simulink model "calculatingcontrol"  (R2023b)
settings: Solver=VariableStepAuto  StartTime=0.0  StopTime=4  RelTol=1e-3
values from neighbouring files (symbols this model uses):
  Kd = params(3)    [ObjectiveFunction_FOPID.m]    (also in run_FOPID_Control.m = best_position_SSA(3))
  Kp = params(1)    [ObjectiveFunction_FOPID.m]    (also in run_FOPID_Control.m = best_position_SSA(1))
undefined symbols (not defined in the file or in its folder): my_gravity_torque, my_mass_matrix, my_velocity_product, q_d, qd_d
settings Model: Creator=孙伟杰  LastModifiedBy=孙伟杰

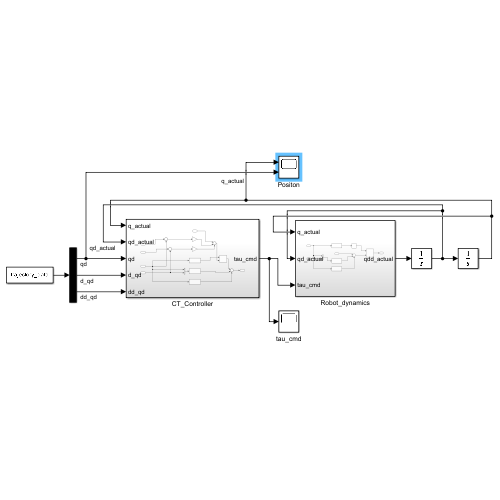
[thumbnail: Simulink's stored preview of the top-level diagram]
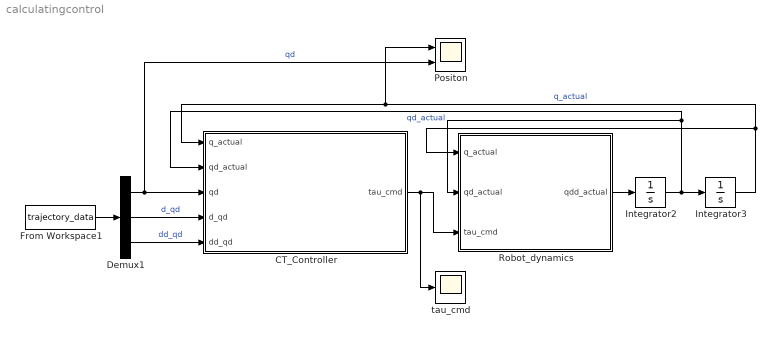
== system calculatingcontrol ==
  CT_Controller : Subsystem
  Demux1 : Demux  Outputs=3
  From Workspace1 : FromWorkspace  VariableName=trajectory_data
  Integrator2 : Integrator  InitialCondition=qd_d(:,1)
  Integrator3 : Integrator  InitialCondition=q_d(:,1)
  Positon : Scope  NumInputPorts=2
  Robot_dynamics : Subsystem
  tau_cmd : Scope
  wires:
  Robot_dynamics/1(qdd_actual) -> Integrator2/1
  CT_Controller/1(tau_cmd) -> tau_cmd/1, Robot_dynamics/3(tau_cmd)
  Demux1/2 -> CT_Controller/4(d_qd)  "d_qd"
  Demux1/3 -> CT_Controller/5(dd_qd)  "dd_qd"
  Demux1/1 -> Positon/2, CT_Controller/3(qd)  "qd"
  From Workspace1/1 -> Demux1/1
  Integrator3/1 -> CT_Controller/1(q_actual), Positon/1, Robot_dynamics/1(q_actual)  "q_actual"
  Integrator2/1 -> Integrator3/1, CT_Controller/2(qd_actual), Robot_dynamics/2(qd_actual)  "qd_actual"

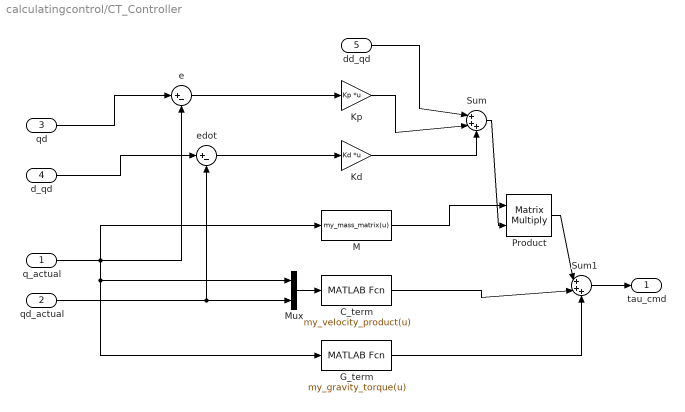
== system calculatingcontrol/CT_Controller ==
  q_actual : Inport
  qd_actual : Inport  Port=2
  qd : Inport  Port=3
  d_qd : Inport  Port=4
  dd_qd : Inport  Port=5
  C_term : MATLABFcn  MATLABFcn=my_velocity_product(u)  OutputDimensions=6
  G_term : MATLABFcn  MATLABFcn=my_gravity_torque(u)  OutputDimensions=6
  Kd : Gain  Gain=Kd  Multiplication=Matrix(K*u) (u vector)
  Kp : Gain  Gain=Kp  Multiplication=Matrix(K*u) (u vector)
  M : MATLABFcn  MATLABFcn=my_mass_matrix(u)  OutputDimensions=[6 6]  Output1D=off
  Mux : Mux  Inputs=2
  Product : Product  Multiplication=Matrix(*)
  Sum : Sum  Inputs=|+++
  Sum1 : Sum  Inputs=|+++
  e : Sum  Inputs=|+-
  edot : Sum  Inputs=|+-
  tau_cmd : Outport
  wires:
  qd/1 -> e/1
  q_actual/1 -> G_term/1, Mux/1, e/2, M/1
  d_qd/1 -> edot/1
  qd_actual/1 -> Mux/2, edot/2
  e/1 -> Kp/1
  edot/1 -> Kd/1
  Mux/1 -> C_term/1
  dd_qd/1 -> Sum/1
  Kp/1 -> Sum/2
  Kd/1 -> Sum/3
  Product/1 -> Sum1/1
  C_term/1 -> Sum1/2
  G_term/1 -> Sum1/3
  Sum1/1 -> tau_cmd/1
  M/1 -> Product/1
  Sum/1 -> Product/2

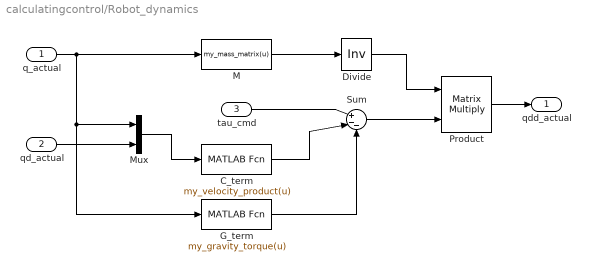
== system calculatingcontrol/Robot_dynamics ==
  q_actual : Inport
  qd_actual : Inport  Port=2
  tau_cmd : Inport  Port=3
  C_term : MATLABFcn  MATLABFcn=my_velocity_product(u)  OutputDimensions=6
  Divide : Product  Inputs=/  Multiplication=Matrix(*)
  G_term : MATLABFcn  MATLABFcn=my_gravity_torque(u)  OutputDimensions=6
  M : MATLABFcn  MATLABFcn=my_mass_matrix(u)  OutputDimensions=[6 6]  Output1D=off
  Mux : Mux  Inputs=2
  Product : Product  Multiplication=Matrix(*)
  Sum : Sum  Inputs=|+--
  qdd_actual : Outport
  wires:
  q_actual/1 -> G_term/1, Mux/1, M/1
  Mux/1 -> C_term/1
  qd_actual/1 -> Mux/2
  tau_cmd/1 -> Sum/1
  C_term/1 -> Sum/2
  G_term/1 -> Sum/3
  M/1 -> Divide/1
  Sum/1 -> Product/2
  Divide/1 -> Product/1
  Product/1 -> qdd_actual/1
